simulink model "BSCU_Brake_cmd"  (Simulink 8.7)
settings: Solver=VariableStepAuto  StartTime=0.0  StopTime=10.0  RelTol=1e-3
values from neighbouring files (symbols this model uses):
  BRAKE_PRESSURE_LO = Simulink.Parameter    [set_up_parameters.m]
  BRAKE_PRESSURE_MAX = Simulink.Parameter    [set_up_parameters.m]
  BRAKE_PRESSURE_MED = Simulink.Parameter    [set_up_parameters.m]
  LO = Simulink.Parameter    [set_up_parameters.m]
  MANUAL = Simulink.Parameter    [set_up_parameters.m]
  MAX = Simulink.Parameter    [set_up_parameters.m]
  MED = Simulink.Parameter    [set_up_parameters.m]
settings Model: Creator=bourbouh  LastModifiedBy=bourbouh
settings DataIOCC: LimitDataPoints=off  SaveFormat=Dataset
settings DebuggingCC: UnderspecifiedInitializationDetection=Simplified  MergeDetectMultiDrivingBlocksExec=error
settings HardwareCC: ProdBitPerPointer=64  ProdLargestAtomicFloat=Float  ProdIntDivRoundTo=Zero  ProdEndianess=LittleEndian  ProdWordSize=64  ProdHWDeviceType=Intel->x86-64 (Windows64)
settings ModelReferenceCC: PropagateSignalLabelsOutOfModel=on
settings ConfigComp: CovModelRefEnable=off

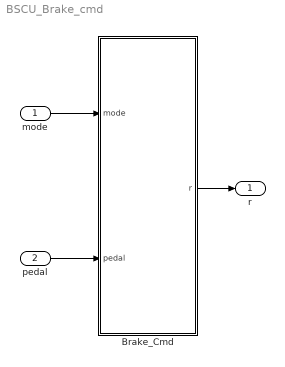
== system BSCU_Brake_cmd ==
  mode : Inport
  pedal : Inport  Port=2
  Brake_Cmd : Stateflow chart  TreatAsAtomicUnit=on
  r : Outport
  wires:
  mode/1 -> Brake_Cmd/1(mode)
  pedal/1 -> Brake_Cmd/2(pedal)
  Brake_Cmd/1(r) -> r/1

== stateflow chart Brake_Cmd ==
  (default) -> (junction 13)
  (junction 13) -> (junction 14) [order 1] : [mode == LO]
  (junction 13) -> (junction 15) [order 2]
  (junction 14) -> (junction 23) : {
      | r = BRAKE_PRESSURE_LO;
      | }
  (junction 15) -> (junction 16) [order 1] : [mode == MED ]
  (junction 15) -> (junction 17) [order 2]
  (junction 16) -> (junction 22) : {
      | r = BRAKE_PRESSURE_MED;
      | }
  (junction 17) -> (junction 18) [order 1] : [mode == MAX]
  (junction 17) -> (junction 19) [order 2]
  (junction 18) -> (junction 21) : {
      | r = BRAKE_PRESSURE_MAX;
      | }
  (junction 19) -> (junction 20) : {
      | r = pedal;
      | }
  (junction 21) -> (junction 20)
  (junction 22) -> (junction 21)
  (junction 23) -> (junction 22)
  (junction 20) -> (junction 24)
  data: mode input int32; pedal input int32; r output int32; MANUAL parameter uint8 =1; LO parameter uint8 =2; MED parameter uint8 =3; MAX parameter uint8 =4; BRAKE_PRESSURE_LO parameter double; BRAKE_PRESSURE_MAX parameter double; BRAKE_PRESSURE_MED parameter double
